simulink model "throttle_sim"  (R2024b)
settings: Solver=VariableStepAuto  StartTime=0.0  StopTime=10.0  RelTol=1e-3
values from neighbouring files (symbols this model uses):
  Cv_F_lower = -1    [run_sim.m]
  Cv_F_upper = 1    [run_sim.m]
  Cv_line = 1    [run_sim.m]
  Cv_OX_lower = -1    [run_sim.m]
  Cv_OX_upper = 1    [run_sim.m]
  F_cmd = 1    [run_sim.m]
  k = 1    [run_sim.m]
  m_F_0 = 1    [run_sim.m]
  m_OX_0 = 1    [run_sim.m]
  omega_c = 1    [run_sim.m]
  P_C_0 = 1    [run_sim.m]
  P_FOX_0 = 1    [run_sim.m]
  P_inf = 1    [run_sim.m]
  R_C = 1    [run_sim.m]
  R_N2 = 1    [run_sim.m]
  rho_F = 1    [run_sim.m]
  rho_H2O = 1    [run_sim.m]
  rho_OX = 1    [run_sim.m]
  T_C = 1    [run_sim.m]
  T_FOX = 1    [run_sim.m]
  Tc = 1    [run_sim.m]
  Ts = 1    [run_sim.m]
  V_C = 1    [run_sim.m]
  V_FOX = 1    [run_sim.m]
  V_plunger = 1    [run_sim.m]
libraries: slpidlib x2, simulink_extras x2, cstblocks x1, simulink x1
settings Model: Creator=devin  LastModifiedBy=devin

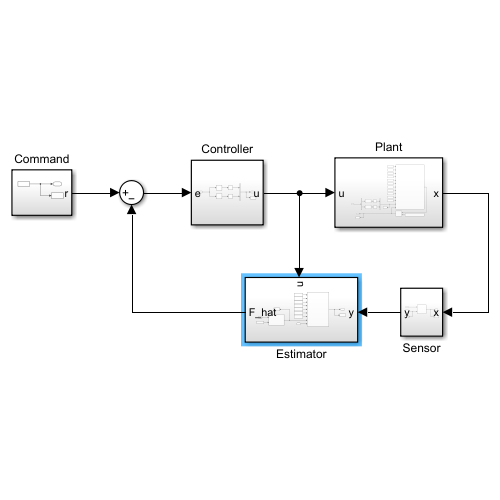
[thumbnail: Simulink's stored preview of the top-level diagram]
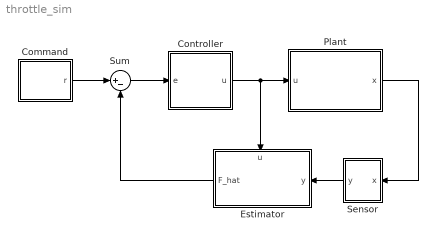
== system throttle_sim ==
  Command : Subsystem
  Controller : Subsystem
  Estimator : Subsystem
      settings: PortSchema="{\"entries\":[{\"content\":{\"sides\":[{\"content\":{\"connectorIds\":[\"In1\"]},\"type\":\"ConnectorPlacement.EquallySpacedRectSide\",\"uuid\":\"20fb6a53-0bbb-41d0-a6d3-dea87dd9b915\"},{\"content\":{\"connectorIds\":[\"Out1\"],\"side\":\"RIGHT\"},\"type\":\"ConnectorPlacement.EquallySpacedRectSide\",\"uuid\":\"d385f8a7-8462-4879-abd9-70f546bdc20b\"},{\"content\":{\"connectorIds\":[\"In2\"],\"side\":\"TOP\"},\"type\":\"ConnectorPlacement.EquallySpacedRectSide\",\"uuid\":\"13e33e7d-6cf2-4b2a-98c6-7b2d337820db\"}]},\"type\":\"ConnectorPlacement.EquallySpacedConnector\",\"uuid\":\"2b346505-005e-4fea-9c00-0780665cb88c\"}],\"packageUris\":[\"http://schema.mathworks.com/mf0/Connector/R2020b\"],\"version\":\"1.0\"}"
  Plant : Subsystem
  Sensor : Subsystem
  Sum : Sum  Inputs=|+-
  wires:
  Plant/1(x) -> Sensor/1(x)
  Sensor/1(y) -> Estimator/1(y)
  Estimator/1(F_hat) -> Sum/2
  Sum/1 -> Controller/1(e)
  Command/1(r) -> Sum/1
  Controller/1(u) -> Plant/1(u), Estimator/2(u)

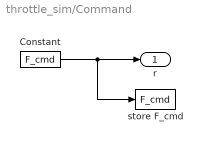
== system throttle_sim/Command ==
  Constant : Constant  Value=F_cmd  SampleTime=Ts
  store F_cmd : ToWorkspace  VariableName=F_cmd  SaveFormat=Timeseries  SampleTime=-1
  r : Outport
  wires:
  Constant/1 -> store F_cmd/1, r/1

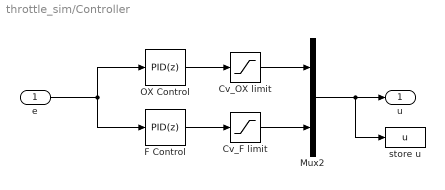
== system throttle_sim/Controller ==
  e : Inport  SampleTime=Tc
  Cv_F limit : Saturate  UpperLimit=Cv_F_upper  LowerLimit=Cv_F_lower
  Cv_OX limit : Saturate  UpperLimit=Cv_OX_upper  LowerLimit=Cv_OX_lower
  F Control : slpidlib/PID Controller  Controller=PID  Form=Parallel  TimeDomain=Discrete-time  UseExternalTs=off  SampleTime=-1  IntegratorMethod=Forward Euler  FilterMethod=Forward Euler  ControllerParametersSource=internal  P=1  I=1  UseKiTs=off  D=0  UseExternalDerivativeSource=off  N=100  UseFilter=on  TunerSelectOption=Transfer Function Based (PID Tuner App)  InitialConditionSource=internal  InitialConditionForIntegrator=0  InitialConditionForFilter=0  DifferentiatorICPrevScaledInput=0  ExternalReset=none  TrackingMode=off  Kt=1  LimitOutput=off  SatLimitsSource=internal  UpperSaturationLimit=inf  LowerSaturationLimit=-inf  LinearizeAsGain=off  AntiWindupMode=none  Kb=1  LimitIntegrator=off  UpperIntegratorSaturationLimit=inf  LowerIntegratorSaturationLimit=-inf  POutMin=[]  POutMax=[]  IOutMin=[]  IOutMax=[]  DOutMin=[]  DOutMax=[]  NOutMin=[]  NOutMax=[]  SumOutMin=[]  SumOutMax=[]  SaturationOutMin=[]  SaturationOutMax=[]  PParamMin=[]  PParamMax=[]  IParamMin=[]  IParamMax=[]  DParamMin=[]  DParamMax=[]  NParamMin=[]  NParamMax=[]  KbParamMin=[]  KbParamMax=[]  KtParamMin=[]  KtParamMax=[]  KbOutMin=[]  KbOutMax=[]  KtOutMin=[]  KtOutMax=[]  IntegratorOutMin=[]  IntegratorOutMax=[]  FilterOutMin=[]  FilterOutMax=[]  SumI1OutMin=[]  SumI1OutMax=[]  SumI2OutMin=[]  SumI2OutMax=[]  SumI3OutMin=[]  SumI3OutMax=[]  SumI4OutMin=[]  SumI4OutMax=[]  SumDOutMin=[]  SumDOutMax=[]  DifferentiatorOutMin=[]  DifferentiatorOutMax=[]  FilterDiffOutCoefMin=[]  FilterDiffOutCoefMax=[]  ReciprocalOutMin=[]  ReciprocalOutMax=[]  SumDenOutMin=[]  SumDenOutMax=[]  SumNumOutMin=[]  SumNumOutMax=[]  DivideOutMin=[]  DivideOutMax=[]  UdiffTsProdOutMin=[]  UdiffTsProdOutMax=[]  NTsProdOutMin=[]  NTsProdOutMax=[]  UintegralTsProdOutMin=[]  UintegralTsProdOutMax=[]  UngainTsProdOutMin=[]  UngainTsProdOutMax=[]  ClampingZeroOutDataTypeStr=Inherit: Inherit via back propagation  ClampingZeroOutMin=[]  ClampingZeroOutMax=[]  FilterDenConstantOutDataTypeStr=Inherit: Inherit via back propagation  FilterDenConstantOutMin=[]  FilterDenConstantOutMax=[]  PCopyOutDataTypeStr=Inherit: Inherit via back propagation  PCopyOutMin=[]  PCopyOutMax=[]  NCopyOutDataTypeStr=Inherit: Inherit via back propagation  NCopyOutMin=[]  NCopyOutMax=[]  IntegratorContinuousStateAttributes=''  IntegratorStateMustResolveToSignalObject=off  IntegratorRTWStateStorageClass=Auto  FilterContinuousStateAttributes=''  FilterStateMustResolveToSignalObject=off  FilterRTWStateStorageClass=Auto  ParallelPVariant=InternalParameters  IdealPVariant=Disabled  IVariant=InternalParameters  DVariant=InternalParameters  IntegratorVariant=Discrete  SatVariant=Disabled  AWVariant=Passthrough  PCopyVariant=Disabled  TRVariant=Disabled  FdbkBlocksVariant=Forward  IdealPFdbkVariant=Disabled  SatFdbkVariant=Disabled  DerivativeFilterVariant=ForwardEulerFilter  NVariant=InternalParameters  NCopyVariant=Disabled  FilterICVariant=InternalICsFilter  IntegratorICVariant=InternalICs  ExternalResetVariant=Disabled  TRSumVariant=Passthrough  SumFdbkVariant=Disabled  SumVariant=Sum_PID  TsampFilterVariant=InternalTs  TsampNgainVariant=Passthrough  TsampIntegralVariant=Disabled_SignalSpec  ExternalSaturationOutDataTypeStr=Inherit: Same as second input  DerivativeSourceVariant=ErrorSignal  PreIntVariant=InternalPreInt
      settings: LibrarySourceBlock=simulink/Discrete/Discrete PID Controller
  Mux2 : Mux  Inputs=2
  OX Control : slpidlib/PID Controller  Controller=PID  Form=Parallel  TimeDomain=Discrete-time  UseExternalTs=off  SampleTime=-1  IntegratorMethod=Forward Euler  FilterMethod=Forward Euler  ControllerParametersSource=internal  P=1  I=1  UseKiTs=off  D=0  UseExternalDerivativeSource=off  N=100  UseFilter=on  TunerSelectOption=Transfer Function Based (PID Tuner App)  InitialConditionSource=internal  InitialConditionForIntegrator=0  InitialConditionForFilter=0  DifferentiatorICPrevScaledInput=0  ExternalReset=none  TrackingMode=off  Kt=1  LimitOutput=off  SatLimitsSource=internal  UpperSaturationLimit=inf  LowerSaturationLimit=-inf  LinearizeAsGain=off  AntiWindupMode=none  Kb=1  LimitIntegrator=off  UpperIntegratorSaturationLimit=inf  LowerIntegratorSaturationLimit=-inf  POutMin=[]  POutMax=[]  IOutMin=[]  IOutMax=[]  DOutMin=[]  DOutMax=[]  NOutMin=[]  NOutMax=[]  SumOutMin=[]  SumOutMax=[]  SaturationOutMin=[]  SaturationOutMax=[]  PParamMin=[]  PParamMax=[]  IParamMin=[]  IParamMax=[]  DParamMin=[]  DParamMax=[]  NParamMin=[]  NParamMax=[]  KbParamMin=[]  KbParamMax=[]  KtParamMin=[]  KtParamMax=[]  KbOutMin=[]  KbOutMax=[]  KtOutMin=[]  KtOutMax=[]  IntegratorOutMin=[]  IntegratorOutMax=[]  FilterOutMin=[]  FilterOutMax=[]  SumI1OutMin=[]  SumI1OutMax=[]  SumI2OutMin=[]  SumI2OutMax=[]  SumI3OutMin=[]  SumI3OutMax=[]  SumI4OutMin=[]  SumI4OutMax=[]  SumDOutMin=[]  SumDOutMax=[]  DifferentiatorOutMin=[]  DifferentiatorOutMax=[]  FilterDiffOutCoefMin=[]  FilterDiffOutCoefMax=[]  ReciprocalOutMin=[]  ReciprocalOutMax=[]  SumDenOutMin=[]  SumDenOutMax=[]  SumNumOutMin=[]  SumNumOutMax=[]  DivideOutMin=[]  DivideOutMax=[]  UdiffTsProdOutMin=[]  UdiffTsProdOutMax=[]  NTsProdOutMin=[]  NTsProdOutMax=[]  UintegralTsProdOutMin=[]  UintegralTsProdOutMax=[]  UngainTsProdOutMin=[]  UngainTsProdOutMax=[]  ClampingZeroOutDataTypeStr=Inherit: Inherit via back propagation  ClampingZeroOutMin=[]  ClampingZeroOutMax=[]  FilterDenConstantOutDataTypeStr=Inherit: Inherit via back propagation  FilterDenConstantOutMin=[]  FilterDenConstantOutMax=[]  PCopyOutDataTypeStr=Inherit: Inherit via back propagation  PCopyOutMin=[]  PCopyOutMax=[]  NCopyOutDataTypeStr=Inherit: Inherit via back propagation  NCopyOutMin=[]  NCopyOutMax=[]  IntegratorContinuousStateAttributes=''  IntegratorStateMustResolveToSignalObject=off  IntegratorRTWStateStorageClass=Auto  FilterContinuousStateAttributes=''  FilterStateMustResolveToSignalObject=off  FilterRTWStateStorageClass=Auto  ParallelPVariant=InternalParameters  IdealPVariant=Disabled  IVariant=InternalParameters  DVariant=InternalParameters  IntegratorVariant=Discrete  SatVariant=Disabled  AWVariant=Passthrough  PCopyVariant=Disabled  TRVariant=Disabled  FdbkBlocksVariant=Forward  IdealPFdbkVariant=Disabled  SatFdbkVariant=Disabled  DerivativeFilterVariant=ForwardEulerFilter  NVariant=InternalParameters  NCopyVariant=Disabled  FilterICVariant=InternalICsFilter  IntegratorICVariant=InternalICs  ExternalResetVariant=Disabled  TRSumVariant=Passthrough  SumFdbkVariant=Disabled  SumVariant=Sum_PID  TsampFilterVariant=InternalTs  TsampNgainVariant=Passthrough  TsampIntegralVariant=Disabled_SignalSpec  ExternalSaturationOutDataTypeStr=Inherit: Same as second input  DerivativeSourceVariant=ErrorSignal  PreIntVariant=InternalPreInt
      settings: LibrarySourceBlock=simulink/Discrete/Discrete PID Controller
  store u : ToWorkspace  VariableName=u  SaveFormat=Timeseries  SampleTime=-1
  u : Outport
  wires:
  Mux2/1 -> store u/1, u/1
  OX Control/1 -> Cv_OX limit/1
  e/1 -> F Control/1, OX Control/1
  F Control/1 -> Cv_F limit/1
  Cv_OX limit/1 -> Mux2/1
  Cv_F limit/1 -> Mux2/2

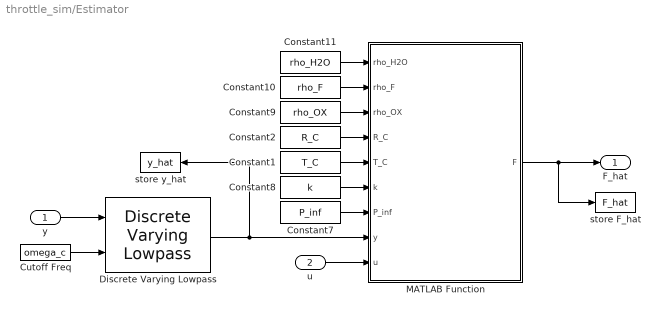
== system throttle_sim/Estimator ==
  y : Inport  SampleTime=Ts
  u : Inport  Port=2  SampleTime=Ts
  Constant1 : Constant  Value=T_C  SampleTime=0
  Constant10 : Constant  Value=rho_F  SampleTime=0
  Constant11 : Constant  Value=rho_H2O  SampleTime=0
  Constant2 : Constant  Value=R_C  SampleTime=0
  Constant7 : Constant  Value=P_inf  SampleTime=0
  Constant8 : Constant  Value=k  SampleTime=0
  Constant9 : Constant  Value=rho_OX  SampleTime=0
  Cutoff Freq : Constant  Value=omega_c  SampleTime=Ts
  Discrete Varying Lowpass : cstblocks/Linear Parameter Varying/Discrete Varying Lowpass  N=1  w0=0  Ts=Ts
  MATLAB Function : MATLAB Function  TreatAsAtomicUnit=on
  store F_hat : ToWorkspace  VariableName=F_hat  SaveFormat=Timeseries  SampleTime=-1
  store y_hat : ToWorkspace  VariableName=y_hat  SaveFormat=Timeseries  SampleTime=-1
  F_hat : Outport
  wires:
  Discrete Varying Lowpass/1 -> store y_hat/1, MATLAB Function/8(y)
  MATLAB Function/1(F) -> store F_hat/1, F_hat/1
  y/1 -> Discrete Varying Lowpass/1
  Cutoff Freq/1 -> Discrete Varying Lowpass/2
  Constant11/1 -> MATLAB Function/1(rho_H2O)
  Constant10/1 -> MATLAB Function/2(rho_F)
  Constant9/1 -> MATLAB Function/3(rho_OX)
  Constant8/1 -> MATLAB Function/6(k)
  Constant7/1 -> MATLAB Function/7(P_inf)
  Constant1/1 -> MATLAB Function/5(T_C)
  Constant2/1 -> MATLAB Function/4(R_C)
  u/1 -> MATLAB Function/9(u)

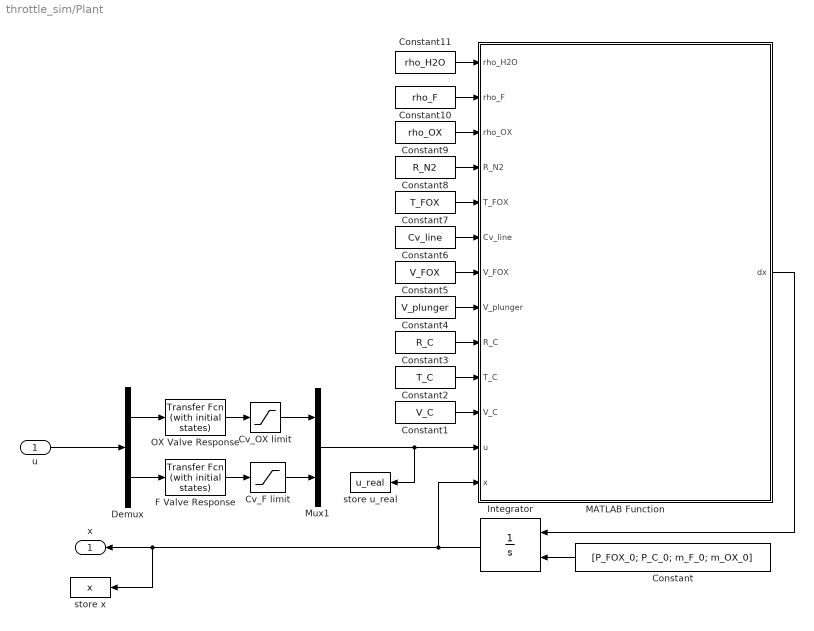
== system throttle_sim/Plant ==
  u : Inport
  Constant : Constant  Value=[P_FOX_0; P_C_0; m_F_0; m_OX_0]  SampleTime=0
  Constant1 : Constant  Value=V_C  SampleTime=0
  Constant10 : Constant  Value=rho_F  SampleTime=0
  Constant11 : Constant  Value=rho_H2O  SampleTime=0
  Constant2 : Constant  Value=T_C  SampleTime=0
  Constant3 : Constant  Value=R_C  SampleTime=0
  Constant4 : Constant  Value=V_plunger  SampleTime=0
  Constant5 : Constant  Value=V_FOX  SampleTime=0
  Constant6 : Constant  Value=Cv_line  SampleTime=0
  Constant7 : Constant  Value=T_FOX  SampleTime=0
  Constant8 : Constant  Value=R_N2  SampleTime=0
  Constant9 : Constant  Value=rho_OX  SampleTime=0
  Cv_F limit : Saturate  UpperLimit=Cv_F_upper  LowerLimit=Cv_F_lower
  Cv_OX limit : Saturate  UpperLimit=Cv_OX_upper  LowerLimit=Cv_OX_lower
  Demux : Demux  Outputs=2
  F Valve Response : simulink_extras/Additional Linear/Transfer Fcn (with initial states)  N=1  D="[1  1]"  X0=0
  Integrator : Integrator  InitialConditionSource=external
  MATLAB Function : MATLAB Function  TreatAsAtomicUnit=on
  Mux1 : Mux  Inputs=2
  OX Valve Response : simulink_extras/Additional Linear/Transfer Fcn (with initial states)  N=[1]  D="[1  1]"  X0=0
  store u_real : ToWorkspace  VariableName=u_real  SaveFormat=Timeseries  SampleTime=-1
  store x : ToWorkspace  VariableName=x  SaveFormat=Timeseries  SampleTime=-1
  x : Outport
  wires:
  MATLAB Function/1(dx) -> Integrator/1
  Mux1/1 -> MATLAB Function/12(u), store u_real/1
  Constant/1 -> Integrator/2
  Demux/2 -> F Valve Response/1
  Demux/1 -> OX Valve Response/1
  u/1 -> Demux/1
  F Valve Response/1 -> Cv_F limit/1
  Cv_F limit/1 -> Mux1/2
  OX Valve Response/1 -> Cv_OX limit/1
  Cv_OX limit/1 -> Mux1/1
  Constant1/1 -> MATLAB Function/11(V_C)
  Constant2/1 -> MATLAB Function/10(T_C)
  Constant3/1 -> MATLAB Function/9(R_C)
  Constant4/1 -> MATLAB Function/8(V_plunger)
  Constant5/1 -> MATLAB Function/7(V_FOX)
  Constant6/1 -> MATLAB Function/6(Cv_line)
  Constant7/1 -> MATLAB Function/5(T_FOX)
  Constant8/1 -> MATLAB Function/4(R_N2)
  Constant9/1 -> MATLAB Function/3(rho_OX)
  Constant10/1 -> MATLAB Function/2(rho_F)
  Constant11/1 -> MATLAB Function/1(rho_H2O)
  Integrator/1 -> MATLAB Function/13(x), x/1, store x/1

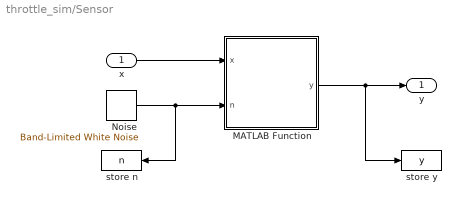
== system throttle_sim/Sensor ==
  x : Inport  SampleTime=Ts
  MATLAB Function : MATLAB Function  TreatAsAtomicUnit=on
  Noise : simulink/Sources/Band-Limited White Noise  Cov=[0.1]  Ts=Ts  seed=[23341]
  store n : ToWorkspace  VariableName=n  SaveFormat=Timeseries  SampleTime=-1
  store y : ToWorkspace  VariableName=y  SaveFormat=Timeseries  SampleTime=-1
  y : Outport
  wires:
  x/1 -> MATLAB Function/1(x)
  MATLAB Function/1(y) -> store y/1, y/1
  Noise/1 -> store n/1, MATLAB Function/2(n)

== matlab function throttle_sim/Sensor/MATLAB Function ==
  data: x input; y output; n input
function y = Measurement(x, n)

% measure P_FOX and P_C
y = x(1:2) + n;

== matlab function throttle_sim/Plant/MATLAB Function ==
  data: rho_H2O input; rho_F input; rho_OX input; R_N2 input; T_FOX input; Cv_line input; V_FOX input; V_plunger input; R_C input; T_C input; V_C input; u input; dx output; x input
function dx = EngineDynamics(rho_H2O, rho_F, rho_OX, R_N2, T_FOX, Cv_line, V_FOX, V_plunger, R_C, T_C, V_C, u, x)

% control variables
Cv_F = u(1);
Cv_OX = u(2);

% state variables
P_FOX = x(1);
P_C = x(2);
m_F = x(3);
m_OX = x(4);

% sqrt terms found in nonlinear equations
sqrt_F  = sqrt((P_FOX - P_C)*rho_H2O*rho_F);
sqrt_OX = sqrt((P_FOX - P_C)*rho_H2O*rho_OX);

% terms for dP_FOX
num1 = R_N2*T_FOX*Cv_line/(V_FOX-V_plunger-m_F/rho_F-m_OX/rho_OX);
num2 = sqrt((1000*6894.76 - P_FOX)*rho_H2O*P_FOX/(R_N2*T_FOX));

% state derivatives
dP_FOX = num1*num2;
dP_C = (Cv_F*sqrt_F + Cv_OX*sqrt_OX)*R_C*T_C/V_C;
dm_F = Cv_F*sqrt_F;
dm_OX = Cv_OX*sqrt_OX;

% dx
dx = [dP_FOX; dP_C; dm_F; dm_OX];

== matlab function throttle_sim/Estimator/MATLAB Function ==
  data: rho_H2O input; rho_F input; rho_OX input; R_C input; T_C input; k input; P_inf input; y input; F output; u input
function F = ThrustCalculation(rho_H2O, rho_F, rho_OX, R_C, T_C, k, P_inf, y, u)

% control variables
Cv_OX = u(1);
Cv_F = u(2);

% state variables
P_FOX = y(1);
P_C = y(2);

% sqrt terms found in nonlinear equations
sqrt_F  = sqrt((P_FOX - P_C)*rho_H2O*rho_F);
sqrt_OX = sqrt((P_FOX - P_C)*rho_H2O*rho_OX);

% terms for F equation
num1 = Cv_F*sqrt_F + Cv_OX*sqrt_OX;
num2 = sqrt(2*k/(k-1)*R_C*T_C*(1-(P_inf/P_C)^((k-1)/k)));

% F
F = num1*num2;
